simulink model "washingmachinecycle"  (R2022a)
settings: Solver=VariableStepAuto  StartTime=0.0  StopTime=85.0  RelTol=1e-3
settings Model: Creator=Amogh  LastModifiedBy=Amogh

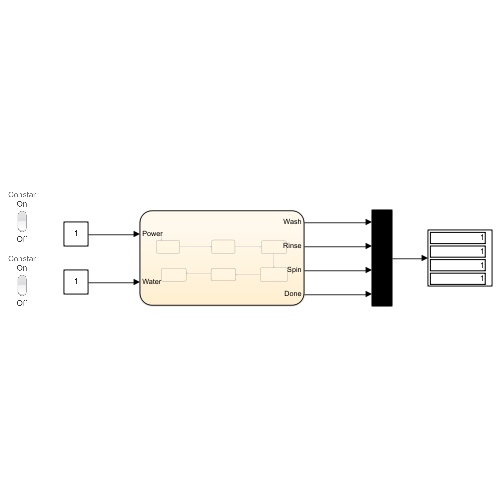
[thumbnail: Simulink's stored preview of the top-level diagram]
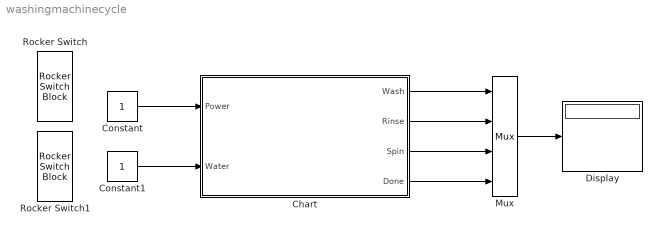
== system washingmachinecycle ==
  Chart : Stateflow chart  TreatAsAtomicUnit=on
  Constant : Constant
  Constant1 : Constant
  Display : Display
  Mux : Mux
  Rocker Switch : RockerSwitchBlock
      settings: Values={{'Off', 'On'}, [0 1]}
  Rocker Switch1 : RockerSwitchBlock
      settings: Values={{'Off', 'On'}, [0 1]}
  wires:
  Constant/1 -> Chart/1(Power)
  Constant1/1 -> Chart/2(Water)
  Mux/1 -> Display/1
  Chart/1(Wash) -> Mux/1
  Chart/2(Rinse) -> Mux/2
  Chart/3(Spin) -> Mux/3
  Chart/4(Done) -> Mux/4

== stateflow chart washingmachinecycle/Chart ==
  state Water
  state Power
  state Wash
    entry:
    Wash=1;
  state Rinse
    entry:
    Rinse=1;
  state Done
    entry:
    Done=1;
  state Spin
    entry:
    Spin=1;
  (default) -> Power
  Power -> Water : [Power==1||after(5,sec)]
  Water -> Wash : [Water==1||after(10,sec)]
  Wash -> Rinse : after(25,sec)
  Spin -> Done : after(20,sec)
  Rinse -> Spin : after(15,sec)
  data: Power input; Water input; Wash output; Rinse output; Spin output; Done output
